simulink library "vmc"  (R2021b)
settings: Solver=VariableStepAuto  StartTime=0.0  StopTime=10.0  RelTol=1e-3
undefined symbols (not defined in the file or in its folder): AVMC_ACCDeltaTqIGain4OVRD_X_kph, AVMC_ACCDeltaTqIGain4OVRD_Y_mps2, AVMC_ACCDeltaTqIGain_X_kph, AVMC_ACCDeltaTqIGain_Y_mps2, AVMC_ACCDeltaTqPGain_X_kph, AVMC_ACCDeltaTqPGain_Y_kph, AVMC_ACCLongSteadyCtrl_X_kph, AVMC_ADSPosGFBDeltaTq_X_kph, AVMC_ADSPosGFBDeltaTq_Y_mps2, AVMC_AggressJerkPCT4AT_X_kph, AVMC_AggressJerkPCT_X_kph, AVMC_AggressLimitPCT4AT_X_kph, AVMC_AggressLimitPCT_X_kph, AVMC_CCLongSteadyCtrl_X_kph, AVMC_DISCDeltaTqIGain_X_kph, AVMC_DISCDeltaTqIGain_Y_mps2, AVMC_DISCDeltaTqPGain_X_kph, AVMC_DISCDeltaTqPGain_Y_kph, AVMC_ESCRegenOut_X_kph, AVMC_ESCRegenOut_Y_Deg, AVMC_ESCRegenOutEnSpd_X_Deg, AVMC_ISOAccLimit_X_mps, AVMC_ISODecLimit_X_mps, AVMC_ISOJerk_X_mps, AVMC_LatESCRegenOut_X_kph, AVMC_LatESCRegenOut_Y_Deg, AVMC_LongAccDeadZone_X_kph, AVMC_LongAccFiltTsforP2_X_Gps, AVMC_MCPresBaseTq_X_bar, AVMC_MSALongSteadyCtrl_X_kph, AVMC_MSAPedalOvrd_X_kph, AVMC_MSASpdBand_X_kph, AVMC_MSATqDownEndTq_X_kph, AVMC_MSATqDownTime_X_kph, AVMC_OPDDisSlideRate_X_Deg, AVMC_OVRD2ActSR2FCMCMD_X_mps2, AVMC_PedalTqRWhlRatio_X_Nm, AVMC_PedalTqRWhlRatio_Y_gps, AVMC_PedalTqRWhlSlipGain_X_rat, AVMC_PedalTqRWhlSlipGain_Y_kph, AVMC_PedalTqRWhSTRGGain_X_deg, AVMC_PedalTqRWhSTRGGain_Y_kph, AVMC_RDCDetectTime_X_kph, AVMC_RDCDetectTime_Y_pct, AVMC_RDCEnSlideRate_X_Deg, AVMC_RearWhlTqRatio_X_Nm, AVMC_RearWhlTqRatio_Y_gps, AVMC_RearWhlTqSlipGain_X_rat, AVMC_RearWhlTqSlipGain_Y_kph, AVMC_RearWhlTqSTRGGain_X_deg, AVMC_RearWhlTqSTRGGain_Y_kph, AVMC_ReqBrkJoinDecSR_X_mps2, AVMC_SoftJerkPCT_X_kph, AVMC_SoftLimitPCT_X_kph, AVMC_StESCYaw_X_kph, AVMC_StESCYaw_Y_Deg, AVMC_StESCYawCom_X_kph, AVMC_StESCYawCom_Y_Gps, AVMC_TMSpdBaseTq_X_rpm, AVMC_VehHoldDecCtrlTime2_X_kph ... (+405)
libraries: hcu_lib x105, simulink x75, tqr x1, simulink_extras x1
(part 4 of 14)

== system vmc/VMC/VMC/MSA function ==
  VTQD_ExternalTqAllow_flg : Inport
  VTQD_DriverWhlTqDem_Nm : Inport  Port=2
  <VTQD_SpdCtrlMode_enum> : Inport  Port=3
  VTQD_SWC2CANCELSta_flg : Inport  Port=4
  VINP_VehSpeed_kph : Inport  Port=5
  VVMC_LongAcc_Gps : Inport  Port=6
  VVMC_FeatSetSpdForCalcu_kph : Inport  Port=7
  VVMC_FeatArbitrFinal_enum : Inport  Port=8
  VTQD_SWC2ResUpSta_flg : Inport  Port=9
  VTQD_SWC2SetdownSta_flg : Inport  Port=10
  VVMC_MeterIndSpeedForCalcu_kph : Inport  Port=11
  VTQD_LowIdleAccPedal_flg : Inport  Port=12
  VDHP_ActAPSPosn_pct : Inport  Port=13
  task_time_s : Inport  Port=14
  VVMC_ActACCRequiredAccel_mps2 : Inport  Port=15
  VTQR_FrTMTqReq_Nm : Inport  Port=16
  VTQR_RrTMTqReq_Nm : Inport  Port=17
  VVMC_TotalAvailBrkRgnTq_Nm : Inport  Port=18
  VINP_HoodSW_flg : Inport  Port=19
  VTQD_GearActualPosn_enum : Inport  Port=20
  VINP_Distanceunit_flg : Inport  Port=21
  VINP_SmartEcoModeSW_flg : Inport  Port=22
  VVMC_APSActive_flg : Inport  Port=23
  VVMC_VMCMSACtrlAvail_flg : Inport  Port=24
  VINP_SWCType_enum : Inport  Port=25
  VTQD_SWC1CANCELSta_flg : Inport  Port=26
  VTQD_SWC1ResUpSta_flg : Inport  Port=27
  VTQD_SWC1SetdownSta_flg : Inport  Port=28
  VVMC_FeatSetSpdFinal_raw32 : Inport  Port=29
  " 2" : Constant  Value=ENUM_SWCTYPE_SWC2
  Add : Sum  Inputs=+-
  Anti-Speed Limitation : Subsystem
  Constant : Constant  Value=TRUE
  Constant1 : Constant  Value=KVMC_CCMSASpdWar_kph
  Constant3 : Constant  Value=ENUM_ADASMSASTA_OFF
  Constant6 : Constant  Value=ENUM_EXTRAMSACTRLSTA_ANTISPEEDLIMIT
  Constant7 : Constant  Value=ENUM_EXTRAMSACTRLSTA_OFF
  Data Type Conversion : DataTypeConversion  OutDataTypeStr=single
  MSAActivationHandshake : Subsystem
  MSADemandTorqueCalculation : Subsystem
  MSATorqueSourceDetermination : Subsystem
  Relational Operator : RelationalOperator  OutDataTypeStr=boolean  RndMeth=Simplest
  Relational Operator3 : RelationalOperator  Operator===  OutDataTypeStr=boolean  RndMeth=Simplest
  Switch{,1..6} (7 alike) : Switch  Criteria=u2 > Threshold
  Unit Delay : UnitDelay  SampleTime=-1  HasFrameUpgradeWarning=on
  VVMC_MSACtrlSta_enum : Outport
  VVMC_MSAWhlTqReq_Nm : Outport  Port=2
  VVMC_MSASpdWar_flg : Outport  Port=3
  VVMC_MSAActive_flg : Outport  Port=4
  VVMC_MSAWhlTqActive_flg : Outport  Port=5
  VVMC_ExtraMSACtrlSta_enum : Outport  Port=6
  VVMC_AntiLimitSpd_kph : Outport  Port=7
  VVMC_AntiSpdLimSpdEn_flg : Outport  Port=8
  wires:
  [VVMC_MSAWhlTqActive_flg] -> VVMC_MSAWhlTqActive_flg/1
  MSATorqueSourceDetermination/3(VVMC_MSAWhlTqActive_flg) -> [VVMC_MSAWhlTqActive_flg]
  [VVMC_MSAActive_flg] -> MSATorqueSourceDetermination/9(VVMC_MSAActive_flg)
  Unit Delay/1 -> MSAActivationHandshake/9(VVMC_MSAOvrdAllow_flg)
  [VVMC_MSAOvrdAllow_flg] -> Unit Delay/1
  [VVMC_MeterIndSpeedForCalcu_kph] -> MSATorqueSourceDetermination/8(VVMC_MeterIndSpeedForCalcu_kph)
  [VTQD_LowIdleAccPedal_flg] -> MSADemandTorqueCalculation/11(VTQD_LowIdleAccPedal_flg)
  [task_time_s] -> MSADemandTorqueCalculation/10(task_time_s)
  MSATorqueSourceDetermination/2(VVMC_MSAOvrdAllow_flg) -> [VVMC_MSAOvrdAllow_flg]
  [VVMC_MSAOvrdAllow_flg] -> MSADemandTorqueCalculation/9(VVMC_MSAPedalOvrd_flg)
  [VTQR_RrTMTqReq_Nm] -> MSADemandTorqueCalculation/8(VTQR_RrTMTqReq_Nm)
  [VTQR_FrTMTqReq_Nm] -> MSADemandTorqueCalculation/7(VTQR_FrTMTqReq_Nm)
  VTQR_RrTMTqReq_Nm/1 -> [VTQR_RrTMTqReq_Nm]
  VTQR_FrTMTqReq_Nm/1 -> [VTQR_FrTMTqReq_Nm]
  [VVMC_ActACCRequiredAccel_mps2] -> MSADemandTorqueCalculation/6(VVMC_ActACCRequiredAccel_mps2)
  VVMC_ActACCRequiredAccel_mps2/1 -> [VVMC_ActACCRequiredAccel_mps2]
  Switch4/1 -> MSATorqueSourceDetermination/7(VVMC_FeatSetSpdForCalcu_kph)
  [task_time_s] -> MSATorqueSourceDetermination/6(task_time_s)
  task_time_s/1 -> [task_time_s]
  [VINP_VehSpeed_kph] -> MSATorqueSourceDetermination/5(VINP_VehSpeed_kph)
  [VDHP_ActAPSPosn_pct] -> MSATorqueSourceDetermination/4(VDHP_ActAPSPosn_pct)
  [VTQD_LowIdleAccPedal_flg] -> MSATorqueSourceDetermination/3(VTQD_LowIdleAccPedal_flg)
  VTQD_LowIdleAccPedal_flg/1 -> [VTQD_LowIdleAccPedal_flg]
  VDHP_ActAPSPosn_pct/1 -> [VDHP_ActAPSPosn_pct]
  [VVMC_MeterIndSpeedForCalcu_kph] -> MSADemandTorqueCalculation/5(VVMC_MeterIndSpeedForCalcu_kph)
  VVMC_MeterIndSpeedForCalcu_kph/1 -> [VVMC_MeterIndSpeedForCalcu_kph]
  [VVMC_LongAcc_Gps] -> MSADemandTorqueCalculation/4(VVMC_LongAcc_Gps)
  VVMC_LongAcc_Gps/1 -> [VVMC_LongAcc_Gps]
  [VVMC_MeterIndSpeedForCalcu_kph] -> MSAActivationHandshake/4(VVMC_MeterIndSpeedForCalcu_kph)
  [VINP_VehSpeed_kph] -> MSADemandTorqueCalculation/2(VINP_VehSpeed_kph)
  VINP_VehSpeed_kph/1 -> [VINP_VehSpeed_kph]
  [VVMC_MSAActive_flg] -> VVMC_MSAActive_flg/1
  Data Type Conversion/1 -> [VVMC_FeatSetSpdForCalcu_kph]  "VVMC_FeatSetSpdForCalcu_kph"
  [VVMC_MSAWhlTqReq_Nm] -> VVMC_MSAWhlTqReq_Nm/1
  [VVMC_MSASpdWar_flg] -> VVMC_MSASpdWar_flg/1
  [VVMC_MSACtrlSta_enum] -> VVMC_MSACtrlSta_enum/1
  VTQD_DriverWhlTqDem_Nm/1 -> [VTQD_DriverWhlTqDem_Nm]
  VTQD_SWC2CANCELSta_flg/1 -> [VTQD_SWC2CANCELSta_flg]
  VVMC_FeatSetSpdForCalcu_kph/1 -> Data Type Conversion/1
  VTQD_ExternalTqAllow_flg/1 -> [VTQD_ExternalTqAllow_flg]
  VVMC_FeatArbitrFinal_enum/1 -> [VVMC_FeatArbitrFinal_enum]
  [VTQD_DriverWhlTqDem_Nm] -> MSATorqueSourceDetermination/2(VTQD_DriverWhlTqDem_Nm)
  [VVMC_FeatSetSpdForCalcu_kph] -> Switch3/3
  [VTQD_SWC2CANCELSta_flg] -> MSAActivationHandshake/6(VTQD_SWC2CANCELSta_flg)  "VTQD_SWC2CANCELSta_flg"
  [VVMC_FeatSetSpdFinal_raw32] -> MSAActivationHandshake/5(VVMC_FeatSetSpdFinal_raw32)
  [VTQD_ExternalTqAllow_flg] -> MSAActivationHandshake/3(VTQD_ExternalTqAllow_flg)
  [VVMC_FeatArbitrFinal_enum] -> MSAActivationHandshake/2(VVMC_FeatArbitrFinal_enum)
  MSATorqueSourceDetermination/1(VVMC_MSAWhlTqReq_Nm) -> [VVMC_MSAWhlTqReq_Nm]
  [VVMC_MSAWhlTqCal_Nm] -> MSATorqueSourceDetermination/1(VVMC_MSAWhlTqCal_Nm)
  MSADemandTorqueCalculation/1(VVMC_MSAWhlTqCal_Nm) -> [VVMC_MSAWhlTqCal_Nm]
  [VVMC_MSAActive_flg] -> MSADemandTorqueCalculation/3(VVMC_MSAActive_flg)
  Switch/1 -> [VVMC_MSAActive_flg]  "VVMC_MSAActive_flg"
  Switch1/1 -> [VVMC_MSASpdWar_flg]  "VVMC_MSASpdWar_flg"
  Switch2/1 -> [VVMC_MSACtrlSta_enum]  "VVMC_MSACtrlSta_enum"
  <VTQD_SpdCtrlMode_enum>/1 -> [VTQD_SpdCtrlMode_enum]
  [VTQD_SpdCtrlMode_enum] -> MSAActivationHandshake/1(VTQD_SpdCtrlMode_enum)
  VTQD_SWC2SetdownSta_flg/1 -> [VTQD_SWC2SetdownSta_flg]
  VTQD_SWC2ResUpSta_flg/1 -> [VTQD_SWC2ResUpSta_flg]
  [VTQD_SWC2ResUpSta_flg] -> MSAActivationHandshake/7(VTQD_SWC2ResUpSta_flg)  "VTQD_SWC2ResUpSta_flg"
  [VTQD_SWC2SetdownSta_flg] -> MSAActivationHandshake/8(VTQD_SWC2SetdownSta_flg)  "VTQD_SWC2SetdownSta_flg"
  VVMC_TotalAvailBrkRgnTq_Nm/1 -> [VVMC_TotalAvailBrkRgnTq_Nm]
  [VVMC_TotalAvailBrkRgnTq_Nm] -> MSADemandTorqueCalculation/12(VVMC_TotalAvailBrkRgnTq_Nm)
  VINP_HoodSW_flg/1 -> [VINP_HoodSW_flg]
  [VTQD_GearActualPosn_enum] -> Anti-Speed Limitation/2(VTQD_GearActualPosn_enum)
  [VINP_HoodSW_flg] -> Anti-Speed Limitation/1(VINP_HoodSW_flg)
  VTQD_GearActualPosn_enum/1 -> [VTQD_GearActualPosn_enum]
  [VVMC_AntiSpdLimSpdEn_flg] -> Switch/2
  MSAActivationHandshake/3(VVMC_IntMSAActive_flg) -> Switch/3
  Constant/1 -> Switch/1
  Relational Operator/1 -> Switch1/1
  [VVMC_AntiSpdLimSpdEn_flg] -> Switch1/2
  MSAActivationHandshake/2(VVMC_IntMSASpdWar_flg) -> Switch1/3
  [VVMC_MeterIndSpeedForCalcu_kph] -> Add/1
  [VVMC_AntiLimitSpd_kph] -> Add/2
  Add/1 -> Relational Operator/1
  Constant1/1 -> Relational Operator/2
  Constant3/1 -> Switch2/1
  [VVMC_AntiSpdLimStaEn_flg] -> Switch2/2
  MSAActivationHandshake/1(VVMC_IntMSACtrlSta_enum) -> [VVMC_IntMSACtrlSta_enum], Switch2/3
  [VVMC_AntiSpdLimSpdEn_flg] -> Switch3/2
  Switch3/1 -> MSADemandTorqueCalculation/1(VVMC_FeatSetSpdForCalcu_kph)
  [VVMC_AntiLimitSpd_kph] -> Switch3/1
  [VVMC_AntiLimitSpd_kph] -> Switch4/1
  [VVMC_AntiSpdLimSpdEn_flg] -> Switch4/2
  [VVMC_FeatSetSpdForCalcu_kph] -> Switch4/3
  [VVMC_AntiSpdLimSpdEn_flg] -> MSATorqueSourceDetermination/11(VVMC_AntiSpdLimSpdEn_flg)
  [VINP_Distanceunit_flg] -> MSAActivationHandshake/10(VINP_Distanceunit_flg)
  VINP_Distanceunit_flg/1 -> [VINP_Distanceunit_flg]
  [VVMC_AntiSpdLimEn_flg] -> Switch5/2
  Constant6/1 -> Switch5/1
  Constant7/1 -> Switch5/3
  Switch5/1 -> [VVMC_ExtraMSACtrlSta_enum]  "VVMC_ExtraMSACtrlSta_enum"
  [VVMC_ExtraMSACtrlSta_enum] -> VVMC_ExtraMSACtrlSta_enum/1
  VVMC_APSActive_flg/1 -> [VVMC_APSActive_flg]
  VINP_SmartEcoModeSW_flg/1 -> [VINP_SmartEcoModeSW_flg]
  Anti-Speed Limitation/1(VVMC_AntiSpdLimEn_flg) -> [VVMC_AntiSpdLimEn_flg]
  Anti-Speed Limitation/2(VVMC_AntiLimitSpd_kph) -> [VVMC_AntiLimitSpd_kph]
  Anti-Speed Limitation/3(VVMC_AntiSpdLimSpdEn_flg) -> [VVMC_AntiSpdLimSpdEn_flg]
  Anti-Speed Limitation/4(VVMC_AntiSpdLimStaEn_flg) -> [VVMC_AntiSpdLimStaEn_flg]
  [VINP_SmartEcoModeSW_flg] -> Anti-Speed Limitation/3(VINP_SmartEcoModeSW_flg)
  [VVMC_APSActive_flg] -> Anti-Speed Limitation/4(VVMC_APSActive_flg)
  [VVMC_IntMSACtrlSta_enum] -> Anti-Speed Limitation/5(VVMC_IntMSACtrlSta_enum)
  [VVMC_AntiLimitSpd_kph] -> VVMC_AntiLimitSpd_kph/1
  [VVMC_AntiSpdLimSpdEn_flg] -> VVMC_AntiSpdLimSpdEn_flg/1
  [VTQD_GearActualPosn_enum] -> MSAActivationHandshake/11(VTQD_GearActualPosn_enum)
  VVMC_VMCMSACtrlAvail_flg/1 -> [VVMC_VMCMSACtrlAvail_flg]
  [VVMC_VMCMSACtrlAvail_flg] -> MSAActivationHandshake/12(VVMC_VMCMSACtrlAvail_flg)
  VINP_SWCType_enum/1 -> [VINP_SWCType_enum]
  [VINP_SWCType_enum] -> MSAActivationHandshake/13(VINP_SWCType_enum)
  VTQD_SWC1CANCELSta_flg/1 -> [VTQD_SWC1CANCELSta_flg]
  VTQD_SWC1ResUpSta_flg/1 -> [VTQD_SWC1ResUpSta_flg]
  VTQD_SWC1SetdownSta_flg/1 -> [VTQD_SWC1SetdownSta_flg]
  [VTQD_SWC1CANCELSta_flg] -> MSAActivationHandshake/14(VTQD_SWC1CANCELSta_flg)
  [VTQD_SWC1ResUpSta_flg] -> MSAActivationHandshake/15(VTQD_SWC1ResUpSta_flg)
  [VTQD_SWC1SetdownSta_flg] -> MSAActivationHandshake/16(VTQD_SWC1SetdownSta_flg)
  VVMC_FeatSetSpdFinal_raw32/1 -> [VVMC_FeatSetSpdFinal_raw32]
  [VINP_SWCType_enum] -> Relational Operator3/1
  Relational Operator3/1 -> Switch6/2
  [VTQD_SWC2ResUpSta_flg] -> Switch6/1
  " 2"/1 -> Relational Operator3/2
  Switch6/1 -> MSATorqueSourceDetermination/10(VTQD_SWCResUpSta_flg)
  [VTQD_SWC1ResUpSta_flg] -> Switch6/3

== system vmc/VMC/VMC/PreConditionCheck ==
  VINP_DriverSeatBeltCmd_flg : Inport
  VBCM_DrDoorSW_flg : Inport  Port=2
  VTQD_GearActualPosn_enum : Inport  Port=3
  VINP_EPBSta_enum : Inport  Port=4
  VINP_ACCAvail_flg : Inport  Port=5
  VINP_AEBAvail_flg : Inport  Port=6
  VINP_ESCOFFStatus_enum : Inport  Port=7
  VINP_APSStaSystem_enum : Inport  Port=8
  VTQD_ExternalTqAllow_flg : Inport  Port=9
  VVMC_ACCCtrlAvail_flg : Inport  Port=10
  task_time_s : Inport  Port=11
  VDDM_VMCLongCtrlProhibited_flg : Inport  Port=12
  Cast To Single : DataTypeConversion  OutDataTypeStr=boolean
  Constant : Constant  Value=ENUM_DRDOORSW_CLOSE
  Constant1 : Constant  Value=ENUM_GEARACTUALPOSN_D
  Constant10 : Constant  Value=ENUM_APSSTASYSTEM_ACTIVE
  Constant11 : Constant  Value=ENUM_APSSTASYSTEM_REMOTEACTIVE
  Constant12 : Constant  Value=ENUM_EXTERNALTQALLOW_ALLOW
  Constant13 : Constant  Value=ENUM_ACCCTRLALLOW_ALLOW
  Constant14 : Constant  Value=ENUM_DRDOORSW_CLOSE
  Constant15 : Constant  Value=ENUM_GEARACTUALPOSN_D
  Constant16 : Constant  Value=KVMC_APSSWC_flg
  Constant17 : Constant  Value=ENUM_EPBSTA_RELEASED
  Constant18 : Constant  Value=ENUM_EXTERNALTQALLOW_ALLOW
  Constant{19,21,24,27,30} (5 alike) : Constant  Value=TRUE
  Constant{20,23,26,29} (4 alike) : Constant  Value=KVMC_PreCheckAllowTime_s
  Constant{22,25,28,31} (4 alike) : Constant  Value=FALSE
  Constant3 : Constant  Value=ENUM_EPBSTA_RELEASED
  Constant4 : Constant  Value=ENUM_ACCAVAIL_AVAILABLE
  Constant5 : Constant  Value=ENUM_AEBAVAIL_AVAILABLE
  Constant6 : Constant  Value=ENUM_ESCOFFSTATUS_NORMAL
  Constant7 : Constant  Value=ENUM_DRIVERSEATBELTCMD_LAMPOFF
  Constant8 : Constant  Value=ENUM_GEARACTUALPOSN_D
  Constant9 : Constant  Value=ENUM_GEARACTUALPOSN_N
  Logical Operator : Logic  AllPortsSameDT=off  OutDataTypeStr=boolean
  Logical Operator1 : Logic  Inputs=6  AllPortsSameDT=off  OutDataTypeStr=boolean
  Logical Operator2 : Logic  Inputs=3  AllPortsSameDT=off  OutDataTypeStr=boolean
  Logical Operator3 : Logic  Inputs=4  AllPortsSameDT=off  OutDataTypeStr=boolean
  Logical Operator4 : Logic  AllPortsSameDT=off  OutDataTypeStr=boolean
  Logical Operator5 : Logic  Inputs=5  AllPortsSameDT=off  OutDataTypeStr=boolean
  Logical Operator6 : Logic  Operator=OR  AllPortsSameDT=off  OutDataTypeStr=boolean
  NOT{,1..6} (7 alike) : Logic  Operator=NOT  AllPortsSameDT=off  OutDataTypeStr=boolean
  Relational Operator{,1,3..9,12..15,17..18} (15 alike) : RelationalOperator  Operator===  OutDataTypeStr=boolean  RndMeth=Simplest
  Relational Operator10 : RelationalOperator  Operator=~=  OutDataTypeStr=boolean  RndMeth=Simplest
  Relational Operator11 : RelationalOperator  Operator=~=  OutDataTypeStr=boolean  RndMeth=Simplest
  Relational Operator{16,19..21} (4 alike) : RelationalOperator  OutDataTypeStr=boolean  RndMeth=Simplest
  Timer{,1..3} (4 alike) : hcu_lib/Basic_Blocks/Timer
  u2 > 0 : Switch  Criteria=u2 > Threshold
  u2 > 0 (1){,1..3} (4 alike) : Switch  Criteria=u2 > Threshold
  VVMC_VMCACCCtrlAvail_flg : Outport
  VVMC_VMCAEBCtrlAvail_flg : Outport  Port=2
  VVMC_VMCCCCtrlAvail_flg : Outport  Port=3
  VVMC_VMCMSACtrlAvail_flg : Outport  Port=4
  wires:
  [task_time_s] -> Timer3/3
  Constant31/1 -> u2 > 0 (1)3/3
  Relational Operator21/1 -> u2 > 0 (1)3/2
  Timer3/1 -> Relational Operator21/1
  Constant29/1 -> Relational Operator21/2, Timer3/4
  Constant30/1 -> u2 > 0 (1)3/1
  Logical Operator5/1 -> NOT3/1, Timer3/1
  NOT3/1 -> Timer3/2
  u2 > 0 (1)3/1 -> [VVMC_VMCMSACtrlAvail_flg]  "VVMC_VMCMSACtrlAvail_flg"
  u2 > 0 (1)2/1 -> [VVMC_VMCCCCtrlAvail_flg]  "VVMC_VMCCCCtrlAvail_flg"
  NOT2/1 -> Timer2/2
  Logical Operator4/1 -> Timer2/1, NOT2/1
  Constant27/1 -> u2 > 0 (1)2/1
  Constant26/1 -> Timer2/4, Relational Operator20/2
  Timer2/1 -> Relational Operator20/1
  Relational Operator20/1 -> u2 > 0 (1)2/2
  Constant28/1 -> u2 > 0 (1)2/3
  [task_time_s] -> Timer2/3
  u2 > 0 (1)1/1 -> [VVMC_VMCACCCtrlAvail_flg]  "VVMC_VMCACCCtrlAvail_flg"
  [task_time_s] -> Timer1/3
  Constant25/1 -> u2 > 0 (1)1/3
  Relational Operator19/1 -> u2 > 0 (1)1/2
  Timer1/1 -> Relational Operator19/1
  Constant23/1 -> Relational Operator19/2, Timer1/4
  Constant24/1 -> u2 > 0 (1)1/1
  Logical Operator2/1 -> NOT1/1, Timer1/1
  NOT1/1 -> Timer1/2
  task_time_s/1 -> [task_time_s]
  u2 > 0 (1)/1 -> [VVMC_VMCAEBCtrlAvail_flg]  "VVMC_VMCAEBCtrlAvail_flg"
  Logical Operator3/1 -> Timer/1, NOT/1
  NOT/1 -> Timer/2
  Constant21/1 -> u2 > 0 (1)/1
  Constant20/1 -> Relational Operator16/2, Timer/4
  Relational Operator16/1 -> u2 > 0 (1)/2
  Timer/1 -> Relational Operator16/1
  [task_time_s] -> Timer/3
  Constant22/1 -> u2 > 0 (1)/3
  Cast To Single/1 -> Logical Operator1/6
  u2 > 0/1 -> Cast To Single/1
  Constant19/1 -> u2 > 0/3
  Constant16/1 -> u2 > 0/2
  Relational Operator5/1 -> Logical Operator3/3
  Relational Operator7/1 -> Logical Operator3/1
  Logical Operator6/1 -> Logical Operator3/2
  Relational Operator8/1 -> Logical Operator6/1
  Relational Operator9/1 -> Logical Operator6/2
  [VTQD_GearActualPosn_enum] -> Relational Operator9/1  "VTQD_GearActualPosn_enum"
  Constant9/1 -> Relational Operator9/2
  Constant8/1 -> Relational Operator8/2
  [VTQD_GearActualPosn_enum] -> Relational Operator8/1  "VTQD_GearActualPosn_enum"
  Constant7/1 -> Relational Operator7/2
  [VINP_DriverSeatBeltCmd_flg] -> Relational Operator7/1
  VINP_DriverSeatBeltCmd_flg/1 -> [VINP_DriverSeatBeltCmd_flg]
  [VVMC_VMCMSACtrlAvail_flg] -> VVMC_VMCMSACtrlAvail_flg/1
  Relational Operator18/1 -> Logical Operator5/4
  Relational Operator17/1 -> Logical Operator5/3
  Relational Operator15/1 -> Logical Operator5/2
  Relational Operator14/1 -> Logical Operator5/1
  Constant18/1 -> Relational Operator18/2
  [VTQD_ExternalTqAllow_flg] -> Relational Operator18/1
  Constant14/1 -> Relational Operator14/2
  [VBCM_DrDoorSW_flg] -> Relational Operator14/1  "VBCM_DrDoorSW_flg"
  Constant15/1 -> Relational Operator15/2
  [VTQD_GearActualPosn_enum] -> Relational Operator15/1  "VTQD_GearActualPosn_enum"
  Constant17/1 -> Relational Operator17/2
  [VINP_EPBSta_enum] -> Relational Operator17/1  "VINP_EPBSta_enum"
  Relational Operator13/1 -> Logical Operator2/2
  [VVMC_ACCCtrlAvail_flg] -> Relational Operator13/1
  Constant13/1 -> Relational Operator13/2
  VVMC_ACCCtrlAvail_flg/1 -> [VVMC_ACCCtrlAvail_flg]
  [VVMC_VMCCCCtrlAvail_flg] -> VVMC_VMCCCCtrlAvail_flg/1
  Relational Operator12/1 -> Logical Operator4/2
  [VTQD_ExternalTqAllow_flg] -> Relational Operator12/1
  Constant12/1 -> Relational Operator12/2
  VTQD_ExternalTqAllow_flg/1 -> [VTQD_ExternalTqAllow_flg]
  [VVMC_VMCACCCtrlAvail_flg] -> VVMC_VMCACCCtrlAvail_flg/1
  [VVMC_VMCAEBCtrlAvail_flg] -> VVMC_VMCAEBCtrlAvail_flg/1
  Logical Operator1/1 -> Logical Operator2/3, Logical Operator4/1
  Relational Operator4/1 -> Logical Operator2/1
  Logical Operator/1 -> u2 > 0/1
  Relational Operator6/1 -> Logical Operator1/4
  Relational Operator3/1 -> Logical Operator1/3
  Relational Operator1/1 -> Logical Operator1/2
  Relational Operator/1 -> Logical Operator1/1
  Relational Operator11/1 -> Logical Operator/2
  Relational Operator10/1 -> Logical Operator/1
  Constant11/1 -> Relational Operator11/2
  [VINP_APSStaSystem_enum] -> Relational Operator11/1
  Constant10/1 -> Relational Operator10/2
  [VINP_APSStaSystem_enum] -> Relational Operator10/1
  Constant6/1 -> Relational Operator6/2
  [VINP_ESCOFFStatus_enum] -> Relational Operator6/1  "VINP_ESCOFFStatus_enum"
  Constant5/1 -> Relational Operator5/2
  [VINP_AEBAvail_flg] -> Relational Operator5/1  "VINP_AEBAvail_flg"
  Constant4/1 -> Relational Operator4/2
  [VINP_ACCAvail_flg] -> Relational Operator4/1  "VINP_ACCAvail_flg"
  [VINP_EPBSta_enum] -> Relational Operator3/1  "VINP_EPBSta_enum"
  Constant3/1 -> Relational Operator3/2
  [VTQD_GearActualPosn_enum] -> Relational Operator1/1  "VTQD_GearActualPosn_enum"
  Constant1/1 -> Relational Operator1/2
  [VBCM_DrDoorSW_flg] -> Relational Operator/1  "VBCM_DrDoorSW_flg"
  Constant/1 -> Relational Operator/2
  VINP_APSStaSystem_enum/1 -> [VINP_APSStaSystem_enum]
  VINP_ESCOFFStatus_enum/1 -> [VINP_ESCOFFStatus_enum]
  VINP_AEBAvail_flg/1 -> [VINP_AEBAvail_flg]
  VINP_ACCAvail_flg/1 -> [VINP_ACCAvail_flg]
  VINP_EPBSta_enum/1 -> [VINP_EPBSta_enum]
  VTQD_GearActualPosn_enum/1 -> [VTQD_GearActualPosn_enum]
  VBCM_DrDoorSW_flg/1 -> [VBCM_DrDoorSW_flg]
  VDDM_VMCLongCtrlProhibited_flg/1 -> [VDDM_VMCLongCtrlProhibited_flg]
  [VDDM_VMCLongCtrlProhibited_flg] -> NOT4/1
  NOT4/1 -> Logical Operator3/4
  [VDDM_VMCLongCtrlProhibited_flg] -> NOT5/1
  NOT5/1 -> Logical Operator1/5
  [VDDM_VMCLongCtrlProhibited_flg] -> NOT6/1
  NOT6/1 -> Logical Operator5/5

== system vmc/VMC/VMC/RDC Determination ==
  task_time_s : Inport
  VVMC_ActMaxSlideRate_pct : Inport  Port=2
  VTQD_AfterAvailableTqDemFr_Nm : Inport  Port=3
  VTQD_AfterAvailableTqDemRr_Nm : Inport  Port=4
  VINP_ESCActive_flg : Inport  Port=5
  VINP_SASAngle_Deg : Inport  Port=6
  VINP_LatAccel_Gps : Inport  Port=7
  VINP_VehSpeed_kph : Inport  Port=8
  VINP_YawRate_degps : Inport  Port=9
  VINP_RDCActive_enum : Inport  Port=10
  VINP_DIDGetDynoMode_flg : Inport  Port=11
  RWD : Subsystem
  VVMC_RWDRDCActive_enum : Outport
  VVMC_RDCEnSlideRate_pct : Outport  Port=2
  VVMC_ActStESCYaw_degps : Outport  Port=3
  wires:
  [VINP_YawRate_degps] -> RWD/9(VINP_YawRate_degps)
  VTQD_AfterAvailableTqDemFr_Nm/1 -> [VTQD_AfterAvailableTqDemFr_Nm]
  [VTQD_AfterAvailableTqDemRr_Nm] -> RWD/4(VTQD_AfterAvailableTqDemRr_Nm)
  [VINP_RDCActive_enum] -> RWD/10(VINP_RDCActive_enum)
  [VINP_VehSpeed_kph] -> RWD/8(VINP_VehSpeed_kph)
  [VVMC_RWDRDCActive_enum] -> VVMC_RWDRDCActive_enum/1
  [VINP_LatAccel_Gps] -> RWD/7(VINP_LatAccel_Gps)
  [VVMC_ActMaxSlideRate_pct] -> RWD/2(VVMC_ActMaxSlideRate_pct)
  [VINP_SASAngle_Deg] -> RWD/6(VINP_SASAngle_Deg)
  [task_time_s] -> RWD/1(task_time_s)
  [VTQD_AfterAvailableTqDemFr_Nm] -> RWD/3(VTQD_AfterAvailableTqDemFr_Nm)
  [VINP_ESCActive_flg] -> RWD/5(VINP_ESCActive_flg)
  VINP_RDCActive_enum/1 -> [VINP_RDCActive_enum]
  VINP_SASAngle_Deg/1 -> [VINP_SASAngle_Deg]
  VTQD_AfterAvailableTqDemRr_Nm/1 -> [VTQD_AfterAvailableTqDemRr_Nm]
  task_time_s/1 -> [task_time_s]
  VVMC_ActMaxSlideRate_pct/1 -> [VVMC_ActMaxSlideRate_pct]
  VINP_ESCActive_flg/1 -> [VINP_ESCActive_flg]
  VINP_VehSpeed_kph/1 -> [VINP_VehSpeed_kph]
  RWD/1(VVMC_RWDRDCActive_enum) -> [VVMC_RWDRDCActive_enum]
  RWD/2(VVMC_RDCEnSlideRate_pct) -> [VVMC_RDCEnSlideRate_pct]
  RWD/3(VVMC_ActStESCYaw_Dps) -> [VVMC_ActStESCYaw_degps]
  [VVMC_RDCEnSlideRate_pct] -> VVMC_RDCEnSlideRate_pct/1
  [VVMC_ActStESCYaw_degps] -> VVMC_ActStESCYaw_degps/1
  VINP_DIDGetDynoMode_flg/1 -> [VINP_DIDGetDynoMode_flg]
  [VINP_DIDGetDynoMode_flg] -> RWD/11(VINP_DIDGetDynoMode_flg)
  VINP_YawRate_degps/1 -> [VINP_YawRate_degps]  "VINP_YawRate_degps"
  VINP_LatAccel_Gps/1 -> [VINP_LatAccel_Gps]  "VINP_LatAccel_Gps"

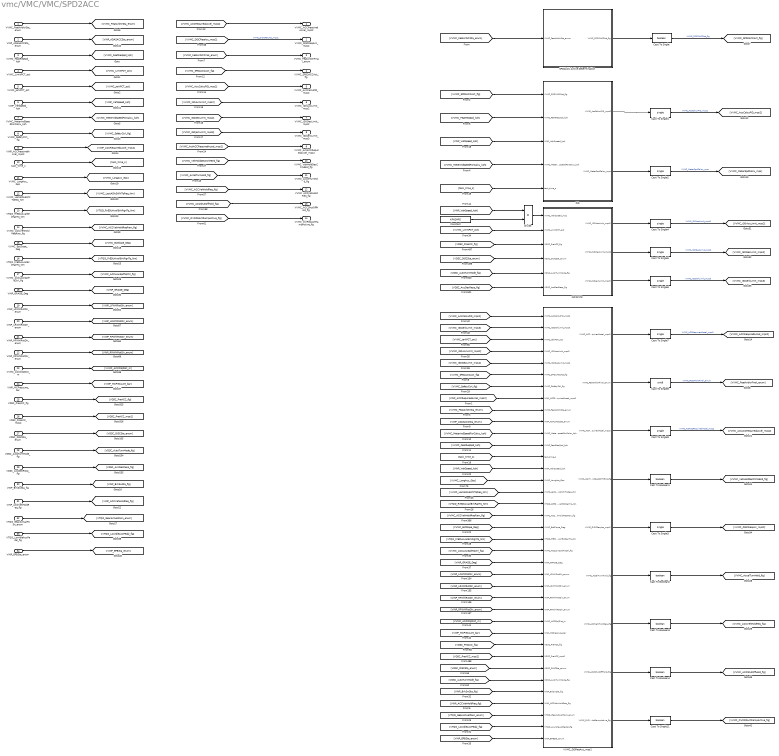
== system vmc/VMC/VMC/SPD2ACC ==
  VVMC_FeatArbitrSta_enum : Inport
  VINP_ADASACCSta_enum : Inport  Port=2
  VVMC_FeatReqSpd_kph : Inport  Port=3
  VVMC_LimitPCT_pct : Inport  Port=4
  VVMC_JerkPCT_pct : Inport  Port=5
  VINP_VehSpeed_kph : Inport  Port=6
  VVMC_MeterIndSpeedForCalcu_kph : Inport  Port=7
  VVMC_SafetyCtrl_flg : Inport  Port=8
  VINP_ACCRequiredAccel_mps2 : Inport  Port=9
  task_time_s : Inport  Port=10
  VVMC_LongAcc_Gps : Inport  Port=11
  VVMC_LastADASWhlTqReq_Nm : Inport  Port=12
  VTQD_RrEDUAvailBrkRgnTq_Nm : Inport  Port=13
  VVMC_ACCVehHoldReqRaw_flg : Inport  Port=14
  VVMC_EstSlope_Deg : Inport  Port=15
  VTQD_FrEDUAvailBrkRgnTq_Nm : Inport  Port=16
  VVMC_ACCLowSpdTqCtrl_flg : Inport  Port=17
  VINP_GRADE_Deg : Inport  Port=18
  VINP_LFWhlRotDir_enum : Inport  Port=19
  VINP_LRWhlRotDir_enum : Inport  Port=20
  VINP_RFWhlRotDir_enum : Inport  Port=21
  VINP_RRWhlRotDir_enum : Inport  Port=22
  VVMC_ACCObjDist_m : Inport  Port=23
  VINP_MCPressure_bar : Inport  Port=24
  VDSC_PreACC_flg : Inport  Port=25
  VDSC_PreACC_mps2 : Inport  Port=26
  VDSC_DISCSta_enum : Inport  Port=27
  VDSC_AutoTurnMode_flg : Inport  Port=28
  VDSC_AccDecResp_flg : Inport  Port=29
  VINP_BrkSwSta_flg : Inport  Port=30
  VINP_ACCVehHoldReq_flg : Inport  Port=31
  VTQD_GearActualPosn_enum : Inport  Port=32
  VTQD_LowIdleAccPedal_flg : Inport  Port=33
  VINP_EPBSta_enum : Inport  Port=34
  Cast To Boolean{1..4} (4 alike) : DataTypeConversion  OutDataTypeStr=boolean
  Cast To Single : DataTypeConversion  OutDataTypeStr=boolean
  Cast To Single{1..7,9} (8 alike) : DataTypeConversion  OutDataTypeStr=single
  Cast To Single11 : DataTypeConversion  OutDataTypeStr=boolean
  Cast To Single8 : DataTypeConversion  OutDataTypeStr=uint8
  Constant : Constant  Value=KPH2MPS
  Divide : Product  Inputs=**
  ISO22179 : Subsystem
  PID : Subsystem
  SPD2ACC Active Determination : Subsystem
  VVMC_DISReqAcc_mps2 : Subsystem
  VVMC_ACCRequiredAccel_mps2 : Outport
  VVMC_DISCReqAcc_mps2 : Outport  Port=2
  VVMC_FeatArbitrFinal_enum : Outport  Port=3
  VVMC_SPD2ACCAct_flg : Outport  Port=4
  VVMC_AccCalcuPID_mps2 : Outport  Port=5
  VVMC_ISOAccLimit_mps2 : Outport  Port=6
  VVMC_ISODecLimit_mps2 : Outport  Port=7
  VVMC_ISOJerkLimit_mps3 : Outport  Port=8
  VVMC_ActACCRequiredAccel_mps2 : Outport  Port=9
  VVMC_VehHoldDecCtrlHEnd_flg : Outport  Port=10
  VVMC_AccelTurnHold_flg : Outport  Port=11
  VVMC_ACCVehHoldReq_flg : Outport  Port=12
  VVMC_ACCShutOffHold_flg : Outport  Port=13
  VVMC_OVRD2ActRampActive_flg : Outport  Port=14
  wires:
  [task_time_s] -> VVMC_DISReqAcc_mps2/13(task_time_s)
  task_time_s/1 -> [task_time_s]
  [VINP_VehSpeed_kph] -> PID/3(VINP_VehSpeed_kph)
  VINP_VehSpeed_kph/1 -> [VINP_VehSpeed_kph]
  [VVMC_ISOJerkLimit_mps3] -> VVMC_ISOJerkLimit_mps3/1
  [VVMC_ISODecLimit_mps2] -> VVMC_ISODecLimit_mps2/1
  [VVMC_ISOAccLimit_mps2] -> VVMC_ISOAccLimit_mps2/1
  [VVMC_AccCalcuPID_mps2] -> VVMC_AccCalcuPID_mps2/1
  [VVMC_SPD2ACCAct_flg] -> VVMC_SPD2ACCAct_flg/1
  [VVMC_FeatReqSpd_kph] -> VVMC_DISReqAcc_mps2/12(VVMC_FeatReqSpd_kph)
  [VVMC_MeterIndSpeedForCalcu_kph] -> VVMC_DISReqAcc_mps2/11(VVMC_MeterIndSpeedForCalcu_kph)
  [VINP_ADASACCSta_enum] -> VVMC_DISReqAcc_mps2/10(VINP_ADASACCSta_enum)
  VINP_ADASACCSta_enum/1 -> [VINP_ADASACCSta_enum]
  [VVMC_DISCReqAcc_mps2] -> VVMC_DISCReqAcc_mps2/1  "VVMC_DISCReqAcc_mps2"
  [VVMC_FeatArbitrFinal_enum] -> VVMC_FeatArbitrFinal_enum/1
  Cast To Single8/1 -> [VVMC_FeatArbitrFinal_enum]  "VVMC_FeatArbitrFinal_enum"
  VVMC_DISReqAcc_mps2/2(VVMC_FeatArbitrFinal_enum) -> Cast To Single8/1
  [VVMC_FeatArbitrSta_enum] -> VVMC_DISReqAcc_mps2/9(VVMC_FeatArbitrSta_enum)
  [VINP_ACCRequiredAccel_mps2] -> VVMC_DISReqAcc_mps2/8(VINP_ACCRequiredAccel_mps2)
  VINP_ACCRequiredAccel_mps2/1 -> [VINP_ACCRequiredAccel_mps2]
  VVMC_SafetyCtrl_flg/1 -> [VVMC_SafetyCtrl_flg]
  [VVMC_SafetyCtrl_flg] -> VVMC_DISReqAcc_mps2/7(VVMC_SafetyCtrl_flg)
  Cast To Single7/1 -> [VVMC_ACCRequiredAccel_mps2]  "VVMC_ACCRequiredAccel_mps2"
  Cast To Single6/1 -> [VVMC_ISOJerkLimit_mps3]  "VVMC_ISOJerkLimit_mps3"
  Cast To Single5/1 -> [VVMC_ISODecLimit_mps2]  "VVMC_ISODecLimit_mps2"
  Cast To Single4/1 -> [VVMC_ISOAccLimit_mps2]  "VVMC_ISOAccLimit_mps2"
  Cast To Single2/1 -> [VVMC_MeterSpdCalcu_mps]  "VVMC_MeterSpdCalcu_mps"
  Cast To Single1/1 -> [VVMC_AccCalcuPID_mps2]  "VVMC_AccCalcuPID_mps2"
  Cast To Single/1 -> [VVMC_SPD2ACCAct_flg]  "VVMC_SPD2ACCAct_flg"
  [VVMC_ACCRequiredAccel_mps2] -> VVMC_ACCRequiredAccel_mps2/1
  VVMC_DISReqAcc_mps2/1("VVMC_ACCRequiredAccel_mps2 ") -> Cast To Single7/1
  [VVMC_SPD2ACCAct_flg] -> VVMC_DISReqAcc_mps2/6(VVMC_SPD2ACCAct_flg)
  PID/2(VVMC_MeterSpdCalcu_mps) -> Cast To Single2/1
  PID/1(VVMC_AccCalcuPID_mps2) -> Cast To Single1/1
  [VVMC_MeterIndSpeedForCalcu_kph] -> PID/4(VVMC_MeterIndSpeedForCalcu_kph)
  [VVMC_SPD2ACCAct_flg] -> PID/1(VVMC_SPD2ACCAct_flg)
  ISO22179/3(VVMC_ISOJerkLimit_mps3) -> Cast To Single6/1
  ISO22179/2(VVMC_ISODecLimit_mps2) -> Cast To Single5/1
  ISO22179/1(VVMC_ISOAccLimit_mps2) -> Cast To Single4/1
  [VVMC_LimitPCT_pct] -> ISO22179/2(VVMC_LimitPCT_pct)
  SPD2ACC Active Determination/1(VVMC_SPD2ACCAct_flg) -> Cast To Single/1
  [VVMC_FeatArbitrSta_enum] -> SPD2ACC Active Determination/1(VVMC_FeatArbitrSta_enum)
  VVMC_FeatArbitrSta_enum/1 -> [VVMC_FeatArbitrSta_enum]
  VVMC_MeterIndSpeedForCalcu_kph/1 -> [VVMC_MeterIndSpeedForCalcu_kph]
  VVMC_LimitPCT_pct/1 -> [VVMC_LimitPCT_pct]
  VVMC_JerkPCT_pct/1 -> [VVMC_JerkPCT_pct]
  VVMC_FeatReqSpd_kph/1 -> [VVMC_FeatReqSpd_kph]
  [VVMC_JerkPCT_pct] -> VVMC_DISReqAcc_mps2/3(VVMC_JerkPCT_pct)
  [VVMC_ISOJerkLimit_mps3] -> VVMC_DISReqAcc_mps2/2(VVMC_ISOJerkLimit_mps3)
  [VVMC_AccCalcuPID_mps2] -> VVMC_DISReqAcc_mps2/1(VVMC_AccCalcuPID_mps2)
  [VVMC_ISOAccLimit_mps2] -> VVMC_DISReqAcc_mps2/4(VVMC_ISOAccLimit_mps2)
  [VVMC_ISODecLimit_mps2] -> VVMC_DISReqAcc_mps2/5(VVMC_ISODecLimit_mps2)
  [VINP_VehSpeed_kph] -> VVMC_DISReqAcc_mps2/14(VINP_VehSpeed_kph)
  [VVMC_LongAcc_Gps] -> VVMC_DISReqAcc_mps2/15(VVMC_LongAcc_Gps)
  VVMC_LongAcc_Gps/1 -> [VVMC_LongAcc_Gps]
  [VTQD_RrEDUAvailBrkRgnTq_Nm] -> VVMC_DISReqAcc_mps2/17(VTQD_RrEDUAvailBrkRgnTq_Nm)
  [VVMC_LastADASWhlTqReq_Nm] -> VVMC_DISReqAcc_mps2/16(VVMC_LastADASWhlTqReq_Nm)
  Cast To Single9/1 -> [VVMC_ActACCRequiredAccel_mps2]  "VVMC_ActACCRequiredAccel_mps2"
  VVMC_DISReqAcc_mps2/3(VVMC_ActACCRequiredAccel_mps2) -> Cast To Single9/1
  VTQD_RrEDUAvailBrkRgnTq_Nm/1 -> [VTQD_RrEDUAvailBrkRgnTq_Nm]
  VVMC_LastADASWhlTqReq_Nm/1 -> [VVMC_LastADASWhlTqReq_Nm]
  [VVMC_ActACCRequiredAccel_mps2] -> VVMC_ActACCRequiredAccel_mps2/1
  VVMC_ACCVehHoldReqRaw_flg/1 -> [VVMC_ACCVehHoldReqRaw_flg]
  [VVMC_ACCVehHoldReqRaw_flg] -> VVMC_DISReqAcc_mps2/18(VVMC_ACCVehHoldReqRaw_flg)
  VVMC_EstSlope_Deg/1 -> [VVMC_EstSlope_Deg]
  [VVMC_EstSlope_Deg] -> VVMC_DISReqAcc_mps2/19(VVMC_EstSlope_Deg)
  VVMC_DISReqAcc_mps2/4(VVMC_VehHoldDecCtrlHEnd_flg) -> Cast To Boolean1/1
  Cast To Boolean1/1 -> [VVMC_VehHoldDecCtrlHEnd_flg]
  [VVMC_VehHoldDecCtrlHEnd_flg] -> VVMC_VehHoldDecCtrlHEnd_flg/1
  VTQD_FrEDUAvailBrkRgnTq_Nm/1 -> [VTQD_FrEDUAvailBrkRgnTq_Nm]
  [VTQD_FrEDUAvailBrkRgnTq_Nm] -> VVMC_DISReqAcc_mps2/20(VTQD_FrEDUAvailBrkRgnTq_Nm)
  VVMC_ACCLowSpdTqCtrl_flg/1 -> [VVMC_ACCLowSpdTqCtrl_flg]
  [VVMC_ACCLowSpdTqCtrl_flg] -> VVMC_DISReqAcc_mps2/21(VVMC_ACCLowSpdTqCtrl_flg)
  VINP_GRADE_Deg/1 -> [VINP_GRADE_Deg]
  [VINP_GRADE_Deg] -> VVMC_DISReqAcc_mps2/22(VINP_GRADE_Deg)
  VINP_LRWhlRotDir_enum/1 -> [VINP_LRWhlRotDir_enum]
  VINP_RFWhlRotDir_enum/1 -> [VINP_RFWhlRotDir_enum]
  VINP_LFWhlRotDir_enum/1 -> [VINP_LFWhlRotDir_enum]
  VINP_RRWhlRotDir_enum/1 -> [VINP_RRWhlRotDir_enum]
  [VINP_RRWhlRotDir_enum] -> VVMC_DISReqAcc_mps2/26(VINP_RRWhlRotDir_enum)
  [VINP_RFWhlRotDir_enum] -> VVMC_DISReqAcc_mps2/25(VINP_RFWhlRotDir_enum)
  [VINP_LRWhlRotDir_enum] -> VVMC_DISReqAcc_mps2/24(VINP_LRWhlRotDir_enum)
  [VINP_LFWhlRotDir_enum] -> VVMC_DISReqAcc_mps2/23(VINP_LFWhlRotDir_enum)
  VVMC_ACCObjDist_m/1 -> [VVMC_ACCObjDist_m]
  [VVMC_ACCObjDist_m] -> VVMC_DISReqAcc_mps2/27(VVMC_ACCObjDist_m)
  VINP_MCPressure_bar/1 -> [VINP_MCPressure_bar]
  [VINP_MCPressure_bar] -> VVMC_DISReqAcc_mps2/28(VINP_MCPressure_bar)
  VVMC_DISReqAcc_mps2/5(VVMC_DISCReqAcc_mps2) -> Cast To Single3/1
  Cast To Single3/1 -> [VVMC_DISCReqAcc_mps2]
  [VVMC_FeatReqSpd_kph] -> PID/2(VVMC_FeatReqSpd_kph)
  Divide/1 -> ISO22179/1(VVMC_VehSpeed_mps)
  [VINP_VehSpeed_kph] -> Divide/1
  Constant/1 -> Divide/2
  [VDSC_PreACC_flg] -> ISO22179/3(VDSC_PreACC_flg)
  [VDSC_DISCSta_enum] -> ISO22179/4(VDSC_DISCSta_enum)
  [VDSC_AutoTurnMode_flg] -> ISO22179/5(VDSC_AutoTurnMode_flg)
  [VDSC_AccDecResp_flg] -> ISO22179/6(VDSC_AccDecResp_flg)
  [VDSC_PreACC_flg] -> VVMC_DISReqAcc_mps2/29(VDSC_PreACC_flg)
  [VDSC_PreACC_mps2] -> VVMC_DISReqAcc_mps2/30(VDSC_PreACC_mps2)
  [VDSC_DISCSta_enum] -> VVMC_DISReqAcc_mps2/31(VDSC_DISCSta_enum)
  [VDSC_AutoTurnMode_flg] -> VVMC_DISReqAcc_mps2/32(VDSC_AutoTurnMode_flg)
  VDSC_AccDecResp_flg/1 -> [VDSC_AccDecResp_flg]
  VDSC_AutoTurnMode_flg/1 -> [VDSC_AutoTurnMode_flg]
  VDSC_DISCSta_enum/1 -> [VDSC_DISCSta_enum]
  VDSC_PreACC_flg/1 -> [VDSC_PreACC_flg]
  VDSC_PreACC_mps2/1 -> [VDSC_PreACC_mps2]
  [VINP_BrkSwSta_flg] -> VVMC_DISReqAcc_mps2/33(VINP_BrkSwSta_flg)
  [VINP_ACCVehHoldReq_flg] -> VVMC_DISReqAcc_mps2/34(VINP_ACCVehHoldReq_flg)
  [VTQD_GearActualPosn_enum] -> VVMC_DISReqAcc_mps2/35(VTQD_GearActualPosn_enum)
  [VTQD_LowIdleAccPedal_flg] -> VVMC_DISReqAcc_mps2/36(VTQD_LowIdleAccPedal_flg)
  [VINP_EPBSta_enum] -> VVMC_DISReqAcc_mps2/37(VINP_EPBSta_enum)
  VTQD_LowIdleAccPedal_flg/1 -> [VTQD_LowIdleAccPedal_flg]
  VINP_BrkSwSta_flg/1 -> [VINP_BrkSwSta_flg]
  VINP_EPBSta_enum/1 -> [VINP_EPBSta_enum]
  VTQD_GearActualPosn_enum/1 -> [VTQD_GearActualPosn_enum]
  VINP_ACCVehHoldReq_flg/1 -> [VINP_ACCVehHoldReq_flg]
  VVMC_DISReqAcc_mps2/8(VVMC_ACCShutOffHold_flg) -> Cast To Boolean4/1
  VVMC_DISReqAcc_mps2/7(VVMC_ACCVehHoldReq_flg) -> Cast To Boolean3/1
  VVMC_DISReqAcc_mps2/6(VVMC_AccelTurnHold_flg) -> Cast To Boolean2/1
  Cast To Boolean2/1 -> [VVMC_AccelTurnHold_flg]
  Cast To Boolean3/1 -> [VVMC_ACCVehHoldReq_flg]
  Cast To Boolean4/1 -> [VVMC_ACCShutOffHold_flg]
  [VVMC_AccelTurnHold_flg] -> VVMC_AccelTurnHold_flg/1
  [VVMC_ACCVehHoldReq_flg] -> VVMC_ACCVehHoldReq_flg/1
  [VVMC_ACCShutOffHold_flg] -> VVMC_ACCShutOffHold_flg/1
  Cast To Single11/1 -> [VVMC_OVRD2ActRampActive_flg]
  VVMC_DISReqAcc_mps2/9(VVMC_OVRD2ActRampActive_flg) -> Cast To Single11/1
  [VVMC_OVRD2ActRampActive_flg] -> VVMC_OVRD2ActRampActive_flg/1
  [task_time_s] -> PID/5(task_time_s)

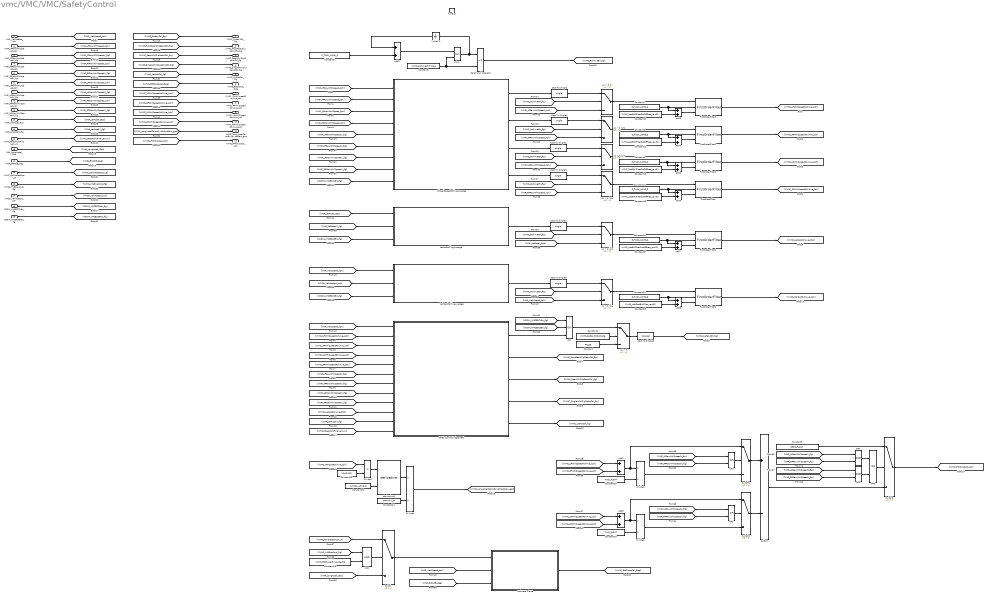
== system vmc/VMC/VMC/SafetyControl ==
  VINP_VehSpeed_kph : Inport
  VINP_LFRawWhlSpeed_kph : Inport  Port=2
  VINP_LFRawWhlSpeedV_flg : Inport  Port=3
  VINP_RFRawWhlSpeed_kph : Inport  Port=4
  VINP_RFRawWhlSpeedV_flg : Inport  Port=5
  VINP_LRRawWhlSpeed_kph : Inport  Port=6
  VINP_LRRawWhlSpeedV_flg : Inport  Port=7
  VINP_RRRawWhlSpeed_kph : Inport  Port=8
  VINP_RRRawWhlSpeedV_flg : Inport  Port=9
  VINP_LatAccel_Gps : Inport  Port=10
  VINP_LatAccelV_flg : Inport  Port=11
  VVMC_FeatArbitrFinal_enum : Inport  Port=12
  VINP_LongAccel_Gps : Inport  Port=13
  VINP_GRADE_deg : Inport  Port=14
  VVMC_CalibratedAccX_G : Inport  Port=15
  VVMC_IMUEnaCmd_flg : Inport  Port=16
  VTQD_VehActSpd_kph : Inport  Port=17
  VDDM_VMCESC1Err_flg : Inport  Port=18
  VDDM_VMCESC5Err_flg : Inport  Port=19
  function : TriggerPort  TriggerType=function-call  VariantControl=(inherit)
  AND : Logic  AllPortsSameDT=off  OutDataTypeStr=boolean
  Add{1..9} (9 alike) : Sum
  Add10 : Sum  Inputs=+-
  Cast To Single{,1..4,8} (6 alike) : DataTypeConversion  OutDataTypeStr=single
  Cast To Single5 : DataTypeConversion  OutDataTypeStr=boolean
  Constant : Constant  Value=FALSE
  Constant1 : Constant  Value=KVMC_SafetyCtrlSWC_flg
  Constant{6..10,16,22,26} (8 alike) : Constant  Value=C_TASK_10MS_S
  Constant{11..13,15} (4 alike) : Constant  Value=KVMC_SpdBWFilterCutOffFreq_raw32
  Constant17 : Constant  Value=KVMC_AccBWFilterCutOffFreq_raw32
  Constant18 : Constant  Value=TWO_FLOAT
  Constant19 : Constant  Value=TWO_FLOAT
  Constant2 : Constant  Value=ZERO_FLOAT
  Constant23 : Constant  Value=KVMC_VehSpdBWFilter_raw32
  Constant24 : Constant  Value=GRAVITY_G
  Constant25 : Constant  Value=KPH2MPS
  Constant28 : Constant  Value=KVMC_EstSlopeGxSource_flg
  Constant5 : Constant  Value=KVMC_RollAveEnTime_s
  Divide2 : Product  Inputs=**
  Divide4 : Product  Inputs=*/
  Divide5 : Product  Inputs=*/
  Divide6 : Product  Inputs=*/
  Estimate Slope : Subsystem
  FirstOrderFilter{,1..4,6} (6 alike) : hcu_lib/Basic_Blocks/FirstOrderFilter
  LatAccRollingAverage : Subsystem
  Min1 : MinMax  Inputs=2
  OR : Logic  Operator=OR  Inputs=3  AllPortsSameDT=off  OutDataTypeStr=boolean
  OR1 : Logic  Operator=OR  AllPortsSameDT=off  OutDataTypeStr=boolean
  OR2 : Logic  Operator=OR  AllPortsSameDT=off  OutDataTypeStr=boolean
  OR3 : Logic  AllPortsSameDT=off  OutDataTypeStr=boolean
  OR4 : Logic  AllPortsSameDT=off  OutDataTypeStr=boolean
  OR5 : Logic  Operator=OR  AllPortsSameDT=off  OutDataTypeStr=boolean
  Relational Operator : RelationalOperator  OutDataTypeStr=boolean  RndMeth=Simplest
  SafetyControlJudgement : Subsystem
  Switch{,1..3} (4 alike) : Switch  Criteria=u2 > Threshold
  VehSpdRollingAverage : Subsystem
  WheelSpeedRollingAverage : Subsystem
  derivative1 : hcu_lib/Basic_Blocks/derivative
  initial: 0 : UnitDelay  SampleTime=-1  HasFrameUpgradeWarning=on
  u2 > 0 : Switch  Criteria=u2 > Threshold
  u2 > 0 (1){,1..4,6} (6 alike) : Switch  Criteria=u2 > Threshold
  VVMC_SafetyCtrl_flg : Outport
  VVMC_FrontRearSlipRatioCtrl_flg : Outport  Port=2
  VVMC_RearWhlSlipRatioCtrl_flg : Outport  Port=3
  VVMC_SingleWhlSlipRatioCtrl_flg : Outport  Port=4
  VVMC_LatAccCtrl_flg : Outport  Port=5
  VVMC_EstSlope_Deg : Outport  Port=6
  VVMC_LFWhlSpeedRollAve_kph : Outport  Port=7
  VVMC_RFWhlSpeedRollAve_kph : Outport  Port=8
  VVMC_LRWhlSpeedRollAve_kph : Outport  Port=9
  VVMC_RRWhlSpeedRollAve_kph : Outport  Port=10
  VVMC_LongAccelCalcuByVehSpdRaw_gps : Outport  Port=11
  VVMC_FrRrSlipSpd_kph : Outport  Port=12
  wires:
  WheelSpeedRollingAverage/4(VVMC_RRWhlSpeedRollAveRaw_kph) -> Cast To Single3/1
  [VINP_LRRawWhlSpeed_kph] -> WheelSpeedRollingAverage/3(VINP_LRRawWhlSpeed_kph)
  FirstOrderFilter/1 -> [VVMC_RRWhlSpeedRollAve_kph]  "VVMC_RRWhlSpeedRollAve_kph"
  [VVMC_LatAccRollAve_Gps] -> SafetyControlJudgement/10(VVMC_LatAccRollAve_Gps)
  [VVMC_SingleWhlSlipRatioCtrl_flg] -> VVMC_SingleWhlSlipRatioCtrl_flg/1
  VINP_LFRawWhlSpeed_kph/1 -> [VINP_LFRawWhlSpeed_kph]
  SafetyControlJudgement/2(VVMC_FrontRearSlipRatioCtrl_flg) -> [VVMC_FrontRearSlipRatioCtrl_flg]
  SafetyControlJudgement/5(VVMC_LatAccCtrl_flg) -> [VVMC_LatAccCtrl_flg]
  [VINP_RFRawWhlSpeed_kph] -> WheelSpeedRollingAverage/2(VINP_RFRawWhlSpeed_kph)
  WheelSpeedRollingAverage/2(VVMC_RFWhlSpeedRollAveRaw_kph) -> Cast To Single1/1
  FirstOrderFilter3/1 -> [VVMC_LFWhlSpeedRollAve_kph]  "VVMC_LFWhlSpeedRollAve_kph"
  [VINP_LatAccelV_flg] -> SafetyControlJudgement/11(VINP_LatAccelV_flg)
  [VINP_LFRawWhlSpeedV_flg] -> SafetyControlJudgement/6(VINP_LFRawWhlSpeedV_flg)
  VINP_RRRawWhlSpeed_kph/1 -> [VINP_RRRawWhlSpeed_kph]
  [VINP_LatAccel_Gps] -> LatAccRollingAverage/1(VINP_LatAccel_Gps)
  LatAccRollingAverage/1(VVMC_LatAccRollAveRaw_Gps) -> Cast To Single4/1
  VINP_LatAccel_Gps/1 -> [VINP_LatAccel_Gps]
  WheelSpeedRollingAverage/1(VVMC_LFWhlSpeedRollAveRaw_kph) -> Cast To Single/1
  SafetyControlJudgement/4(VVMC_SingleWhlSlipRatioCtrl_flg) -> [VVMC_SingleWhlSlipRatioCtrl_flg]
  [VVMC_LatAccCtrl_flg] -> VVMC_LatAccCtrl_flg/1
  [VINP_RFRawWhlSpeedV_flg] -> SafetyControlJudgement/7(VINP_RFRawWhlSpeedV_flg)
  Constant1/1 -> u2 > 0/2
  VINP_LRRawWhlSpeed_kph/1 -> [VINP_LRRawWhlSpeed_kph]
  FirstOrderFilter4/1 -> [VVMC_LatAccRollAve_Gps]  "VVMC_LatAccRollAve_Gps"
  u2 > 0/1 -> Cast To Single5/1
  [VVMC_RearWhlSlipRatioCtrl_flg] -> VVMC_RearWhlSlipRatioCtrl_flg/1
  VINP_RRRawWhlSpeedV_flg/1 -> [VINP_RRRawWhlSpeedV_flg]
  [VVMC_LRWhlSpeedRollAve_kph] -> SafetyControlJudgement/4(VVMC_LRWhlSpeedRollAve_kph)
  [VINP_RRRawWhlSpeed_kph] -> WheelSpeedRollingAverage/4(VINP_RRRawWhlSpeed_kph)
  [VVMC_RRWhlSpeedRollAve_kph] -> SafetyControlJudgement/5(VVMC_RRWhlSpeedRollAve_kph)
  WheelSpeedRollingAverage/3(VVMC_LRWhlSpeedRollAveRaw_kph) -> Cast To Single2/1
  SafetyControlJudgement/3(VVMC_RearWhlSlipRatioCtrl_flg) -> [VVMC_RearWhlSlipRatioCtrl_flg]
  VINP_LatAccelV_flg/1 -> [VINP_LatAccelV_flg]
  [VINP_LFRawWhlSpeed_kph] -> WheelSpeedRollingAverage/1(VINP_LFRawWhlSpeed_kph)
  VINP_LFRawWhlSpeedV_flg/1 -> [VINP_LFRawWhlSpeedV_flg]
  [VVMC_FeatArbitrFinal_enum] -> SafetyControlJudgement/12(VVMC_FeatArbitrFinal_enum)
  SafetyControlJudgement/1(VVMC_SafetyCtrl_flg) -> OR/3
  [VINP_RRRawWhlSpeedV_flg] -> SafetyControlJudgement/9(VINP_RRRawWhlSpeedV_flg)
  [VINP_LRRawWhlSpeedV_flg] -> SafetyControlJudgement/8(VINP_LRRawWhlSpeedV_flg)
  VVMC_FeatArbitrFinal_enum/1 -> [VVMC_FeatArbitrFinal_enum]
  [VINP_VehSpeed_kph] -> SafetyControlJudgement/1(VINP_VehSpeed_kph)
  VINP_LRRawWhlSpeedV_flg/1 -> [VINP_LRRawWhlSpeedV_flg]
  VINP_VehSpeed_kph/1 -> [VINP_VehSpeed_kph]
  [VVMC_SafetyCtrl_flg] -> VVMC_SafetyCtrl_flg/1
  FirstOrderFilter2/1 -> [VVMC_RFWhlSpeedRollAve_kph]  "VVMC_RFWhlSpeedRollAve_kph"
  [VVMC_LFWhlSpeedRollAve_kph] -> SafetyControlJudgement/2(VVMC_LFWhlSpeedRollAve_kph)
  [VVMC_FrontRearSlipRatioCtrl_flg] -> VVMC_FrontRearSlipRatioCtrl_flg/1
  Cast To Single5/1 -> [VVMC_SafetyCtrl_flg]  "VVMC_SafetyCtrl_flg"
  VINP_RFRawWhlSpeed_kph/1 -> [VINP_RFRawWhlSpeed_kph]
  [VVMC_RFWhlSpeedRollAve_kph] -> SafetyControlJudgement/3(VVMC_RFWhlSpeedRollAve_kph)
  FirstOrderFilter1/1 -> [VVMC_LRWhlSpeedRollAve_kph]  "VVMC_LRWhlSpeedRollAve_kph"
  Constant/1 -> u2 > 0/3
  VINP_RFRawWhlSpeedV_flg/1 -> [VINP_RFRawWhlSpeedV_flg]
  initial: 0/1 -> Add2/1
  Constant5/1 -> Min1/2, Relational Operator/2
  Constant6/1 -> Add2/2
  Add2/1 -> Min1/1
  Relational Operator/1 -> [VVMC_RollAveEn_flg]  "VVMC_RollAveEn_flg"
  u2 > 0 (1)2/1 -> FirstOrderFilter1/1
  u2 > 0 (1)/1 -> FirstOrderFilter3/1
  [VINP_RFRawWhlSpeed_kph] -> u2 > 0 (1)1/3
  [VINP_LRRawWhlSpeed_kph] -> u2 > 0 (1)2/3
  [VVMC_RollAveEn_flg] -> u2 > 0 (1)3/2
  [VVMC_RollAveEn_flg] -> u2 > 0 (1)/2
  [VINP_LFRawWhlSpeed_kph] -> u2 > 0 (1)/3
  Cast To Single/1 -> u2 > 0 (1)/1
  [VINP_RRRawWhlSpeed_kph] -> u2 > 0 (1)3/3
  u2 > 0 (1)1/1 -> FirstOrderFilter2/1
  [VVMC_RollAveEn_flg] -> u2 > 0 (1)1/2
  Cast To Single2/1 -> u2 > 0 (1)2/1
  Cast To Single1/1 -> u2 > 0 (1)1/1
  u2 > 0 (1)3/1 -> FirstOrderFilter/1
  Cast To Single3/1 -> u2 > 0 (1)3/1
  [VVMC_RollAveEn_flg] -> u2 > 0 (1)2/2
  Constant7/1 -> Add3/1, FirstOrderFilter3/2
  Constant8/1 -> FirstOrderFilter2/2, Add4/1
  Constant9/1 -> Add5/1, FirstOrderFilter1/2
  Constant10/1 -> FirstOrderFilter/2, Add6/1
  Add3/1 -> FirstOrderFilter3/3
  Constant11/1 -> Add3/2
  Constant12/1 -> Add4/2
  Add4/1 -> FirstOrderFilter2/3
  Constant13/1 -> Add5/2
  Add5/1 -> FirstOrderFilter1/3
  Constant15/1 -> Add6/2
  Add6/1 -> FirstOrderFilter/3
  [VVMC_RollAveEn_flg] -> u2 > 0 (1)4/2
  Cast To Single4/1 -> u2 > 0 (1)4/1
  [VINP_LatAccel_Gps] -> u2 > 0 (1)4/3
  Add7/1 -> FirstOrderFilter4/3
  Constant17/1 -> Add7/2
  Constant16/1 -> FirstOrderFilter4/2, Add7/1
  u2 > 0 (1)4/1 -> FirstOrderFilter4/1
  Switch/1 -> Estimate Slope/1(VINP_LongAccel_Gps)
  [VINP_GRADE_deg] -> Estimate Slope/3(VINP_GRADE_deg)
  [VINP_VehSpeed_kph] -> Estimate Slope/2(VINP_VehSpeed_kph)
  Estimate Slope/1(VVMC_EstSlopeCal_Deg) -> [VVMC_EstSlopeCal_Deg]
  VINP_LongAccel_Gps/1 -> [VINP_LongAccel_Gps]
  VINP_GRADE_deg/1 -> [VINP_GRADE_deg]
  [VVMC_EstSlopeCal_Deg] -> VVMC_EstSlope_Deg/1
  [VVMC_RRWhlSpeedRollAve_kph] -> VVMC_RRWhlSpeedRollAve_kph/1  "VVMC_RRWhlSpeedRollAve_kph"
  [VVMC_LRWhlSpeedRollAve_kph] -> VVMC_LRWhlSpeedRollAve_kph/1  "VVMC_LRWhlSpeedRollAve_kph"
  [VVMC_RFWhlSpeedRollAve_kph] -> VVMC_RFWhlSpeedRollAve_kph/1  "VVMC_RFWhlSpeedRollAve_kph"
  [VVMC_LFWhlSpeedRollAve_kph] -> VVMC_LFWhlSpeedRollAve_kph/1  "VVMC_LFWhlSpeedRollAve_kph"
  [VINP_VehSpeed_kph] -> VehSpdRollingAverage/1(VINP_VehSpeed_kph)
  Add8/1 -> FirstOrderFilter6/3
  Constant23/1 -> Add8/2
  Constant22/1 -> Add8/1, FirstOrderFilter6/2
  Cast To Single8/1 -> u2 > 0 (1)6/1
  u2 > 0 (1)6/1 -> FirstOrderFilter6/1
  [VINP_VehSpeed_kph] -> u2 > 0 (1)6/3
  [VVMC_RollAveEn_flg] -> u2 > 0 (1)6/2
  FirstOrderFilter6/1 -> [VVMC_VehSpdRollAve_kph]  "VVMC_VehSpdRollAve_kph"
  VehSpdRollingAverage/1(VVMC_VehSpdRollAveRaw_kph) -> Cast To Single8/1
  Constant26/1 -> derivative1/2
  derivative1/1 -> Divide4/1
  Constant24/1 -> Divide4/2
  Constant25/1 -> Divide2/2
  [VVMC_VehSpdRollAve_kph] -> Divide2/1
  Divide2/1 -> derivative1/1
  Divide4/1 -> [VVMC_LongAccelCalcuByVehSpdRaw_gps]  "VVMC_LongAccelCalcuByVehSpdRaw_gps"
  [VVMC_LongAccelCalcuByVehSpdRaw_gps] -> VVMC_LongAccelCalcuByVehSpdRaw_gps/1  "VVMC_LongAccelCalcuByVehSpd_gps"
  [VVMC_LFWhlSpeedRollAve_kph] -> Add1/1
  [VVMC_RFWhlSpeedRollAve_kph] -> Add1/2
  Constant18/1 -> Divide5/2
  [VVMC_LRWhlSpeedRollAve_kph] -> Add9/1
  [VVMC_RRWhlSpeedRollAve_kph] -> Add9/2
  Constant19/1 -> Divide6/2
  Add9/1 -> Switch2/1, Divide6/1
  Add1/1 -> Switch1/1, Divide5/1
  Divide6/1 -> Switch2/3
  Divide5/1 -> Switch1/3
  Switch3/1 -> [VVMC_FrRrSlipSpd_kph]  "VVMC_FrRrSlipSpd_kph"
  [VVMC_FrRrSlipSpd_kph] -> VVMC_FrRrSlipSpd_kph/1
  Min1/1 -> initial: 0/1, Relational Operator/1
  VVMC_CalibratedAccX_G/1 -> [VVMC_CalibratedAccX_G]
  VVMC_IMUEnaCmd_flg/1 -> [VVMC_IMUEnaCmd_flg]
  [VVMC_CalibratedAccX_G] -> Switch/1
  AND/1 -> Switch/2
  [VINP_LongAccel_Gps] -> Switch/3
  Constant28/1 -> AND/2
  [VVMC_IMUEnaCmd_flg] -> AND/1
  [VINP_LFRawWhlSpeedV_flg] -> WheelSpeedRollingAverage/5(VINP_LFRawWhlSpeedV_flg)
  [VINP_RFRawWhlSpeedV_flg] -> WheelSpeedRollingAverage/6(VINP_RFRawWhlSpeedV_flg)
  [VINP_LRRawWhlSpeedV_flg] -> WheelSpeedRollingAverage/7(VINP_LRRawWhlSpeedV_flg)
  [VINP_RRRawWhlSpeedV_flg] -> WheelSpeedRollingAverage/8(VINP_RRRawWhlSpeedV_flg)
  [VINP_LatAccelV_flg] -> LatAccRollingAverage/2(VINP_LatAccelV_flg)
  VTQD_VehActSpd_kph/1 -> [VTQD_VehActSpd_kph]
  VDDM_VMCESC1Err_flg/1 -> [VDDM_VMCESC1Err_flg]
  VDDM_VMCESC5Err_flg/1 -> [VDDM_VMCESC5Err_flg]
  [VDDM_VMCESC1Err_flg] -> WheelSpeedRollingAverage/9(VDDM_VMCESC1Err_flg)
  [VDDM_VMCESC5Err_flg] -> LatAccRollingAverage/3(VDDM_VMCESC5Err_flg)
  [VDDM_VMCESC1Err_flg] -> VehSpdRollingAverage/3(VDDM_VMCESC1Err_flg)
  [VTQD_VehActSpd_kph] -> VehSpdRollingAverage/2(VTQD_VehActSpd_kph)
  [VDDM_VMCESC5Err_flg] -> OR/2
  [VDDM_VMCESC1Err_flg] -> OR/1
  OR/1 -> u2 > 0/1
  OR1/1 -> Switch1/2
  [VINP_LFRawWhlSpeedV_flg] -> OR1/1
  [VINP_RFRawWhlSpeedV_flg] -> OR1/2
  Switch1/1 -> Add10/1
  OR2/1 -> Switch2/2
  Switch2/1 -> Add10/2
  [VINP_LRRawWhlSpeedV_flg] -> OR2/1
  [VINP_RRRawWhlSpeedV_flg] -> OR2/2
  [VINP_RRRawWhlSpeedV_flg] -> OR3/2
  [VINP_LRRawWhlSpeedV_flg] -> OR3/1
  [VINP_RFRawWhlSpeedV_flg] -> OR4/2
  [VINP_LFRawWhlSpeedV_flg] -> OR4/1
  OR4/1 -> OR5/1
  OR3/1 -> OR5/2
  OR5/1 -> Switch3/2
  Add10/1 -> Switch3/3
  Constant2/1 -> Switch3/1
